simulink model "sim_punto1"  (R2021b)
settings: Solver=VariableStepAuto  StartTime=0.0  StopTime=10.0  RelTol=1e-3
values from neighbouring files (symbols this model uses):
  A = [0 1 0 0 0 0 0 0 0 0 0 0 ... (first row only)    [punto1.m]
  B = [0; 0; 0; 0; 0; 0; 0; 0; 0; 0; 0; 1]    [punto1.m]
  C = [1 0 0 0 0 0 0 0 0 0 0 0]    [punto1.m]
  C_states = eye(12)    [punto1.m]
  D_states = [0 0 0 0 0 0 0 0 0 0 0 0]'    [punto1.m]
  K = lqr(A, B, Q, R)    [punto1.m]
  Ts = 0.1    [punto1.m]
  U_max = 15    [punto1.m]
  U_min = -15    [punto1.m]
  Ubar = inv(g) * Ybar    [punto1.m]
  Ubar_disc = inv(gd)*Ybar    [punto1.m]
  Xbar = -inv(A) * B * Ubar    [punto1.m]
  Xbar_disc = (eye(12)- Ad)^-1*Bd*Ubar    [punto1.m]
undefined symbols (not defined in the file or in its folder): Ad, Bd, Cd, K_disc
settings Model: Creator=danie  LastModifiedBy=danie

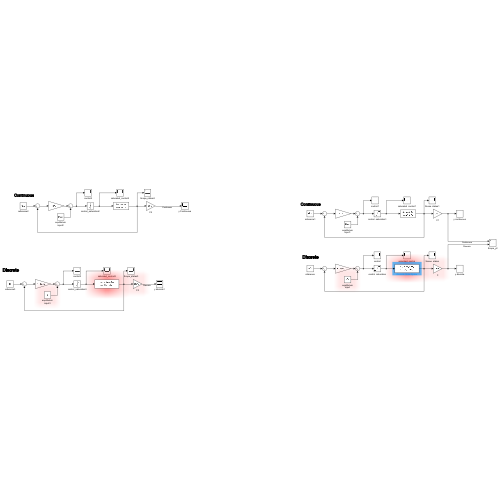
[thumbnail: Simulink's stored preview of the top-level diagram]
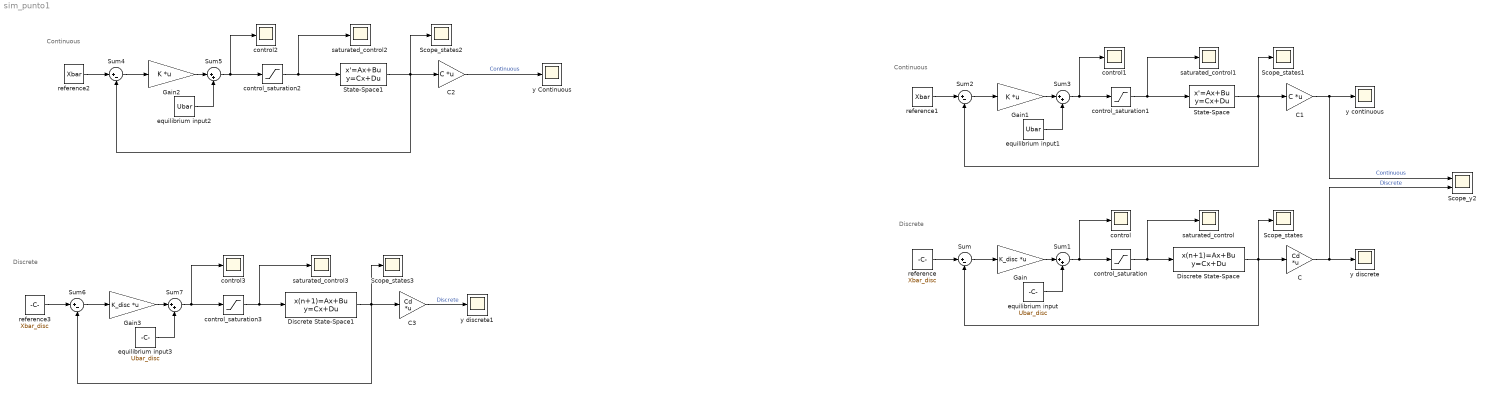
== system sim_punto1 ==
  note: Discrete
  note: Continuous
  note: Continuous
  note: Discrete
  C : Gain  Gain=Cd  Multiplication=Matrix(K*u)
  C1 : Gain  Gain=C  Multiplication=Matrix(K*u)
  C2 : Gain  Gain=C  Multiplication=Matrix(K*u)
  C3 : Gain  Gain=Cd  Multiplication=Matrix(K*u)
  Discrete State-Space : DiscreteStateSpace  A=Ad  B=Bd  C=C_states  D=D_states  SampleTime=Ts
  Discrete State-Space1 : DiscreteStateSpace  A=Ad  B=Bd  C=C_states  D=D_states  SampleTime=Ts
  Gain : Gain  Gain=K_disc  Multiplication=Matrix(K*u)
  Gain1 : Gain  Gain=K  Multiplication=Matrix(K*u)
  Gain2 : Gain  Gain=K  Multiplication=Matrix(K*u)
  Gain3 : Gain  Gain=K_disc  Multiplication=Matrix(K*u)
  Scope_states{,1..3} (4 alike) : Scope
  Scope_y2 : Scope  NumInputPorts=2
  State-Space : StateSpace  A=A  B=B  C=C_states  D=D_states  InitialCondition=0
  State-Space1 : StateSpace  A=A  B=B  C=C_states  D=D_states  InitialCondition=0
  Sum{,2,4,6} (4 alike) : Sum  Inputs=|+-
  Sum{1,3,5,7} (4 alike) : Sum  Inputs=|++
  control{,1..3} (4 alike) : Scope
  control_saturation{,1..3} (4 alike) : Saturate  UpperLimit=U_max  LowerLimit=U_min
  equilibrium input : Constant  Value=Ubar_disc
  equilibrium input1 : Constant  Value=Ubar
  equilibrium input2 : Constant  Value=Ubar
  equilibrium input3 : Constant  Value=Ubar_disc
  reference : Constant  Value=Xbar_disc
  reference1 : Constant  Value=Xbar
  reference2 : Constant  Value=Xbar
  reference3 : Constant  Value=Xbar_disc
  saturated_control{,1..3} (4 alike) : Scope
  y Continuous : Scope
  y continuous : Scope
  y discrete : Scope
  y discrete1 : Scope
  wires:
  reference1/1 -> Sum2/1
  equilibrium input1/1 -> Sum3/2
  Sum3/1 -> control1/1, control_saturation1/1
  C1/1 -> Scope_y2/1, y continuous/1  "Continuous"
  State-Space/1 -> C1/1, Scope_states1/1, Sum2/2
  Sum2/1 -> Gain1/1
  Gain1/1 -> Sum3/1
  control_saturation1/1 -> State-Space/1, saturated_control1/1
  equilibrium input/1 -> Sum1/2
  control_saturation/1 -> Discrete State-Space/1, saturated_control/1
  reference/1 -> Sum/1
  Sum1/1 -> control/1, control_saturation/1
  Discrete State-Space/1 -> C/1, Scope_states/1, Sum/2
  Gain/1 -> Sum1/1
  C/1 -> Scope_y2/2, y discrete/1  "Discrete"
  Sum/1 -> Gain/1
  State-Space1/1 -> C2/1, Scope_states2/1, Sum4/2
  Sum4/1 -> Gain2/1
  Sum5/1 -> control2/1, control_saturation2/1
  reference2/1 -> Sum4/1
  C2/1 -> y Continuous/1  "Continuous"
  control_saturation2/1 -> State-Space1/1, saturated_control2/1
  Gain2/1 -> Sum5/1
  equilibrium input2/1 -> Sum5/2
  Discrete State-Space1/1 -> C3/1, Scope_states3/1, Sum6/2
  C3/1 -> y discrete1/1  "Discrete"
  Sum6/1 -> Gain3/1
  control_saturation3/1 -> Discrete State-Space1/1, saturated_control3/1
  Gain3/1 -> Sum7/1
  equilibrium input3/1 -> Sum7/2
  Sum7/1 -> control3/1, control_saturation3/1
  reference3/1 -> Sum6/1
